simulink model "singlephasesinePWMinverter"  (R2012b)
settings: Solver=ode45  StartTime=0.0  StopTime=1  RelTol=1e-3
libraries: powerlib x7, powerlib_extras x1
settings Model: Creator=Tran Minh Luan  LastModifiedBy=Tran Minh Luan
settings SolverCC: PositivePriorityOrder=on

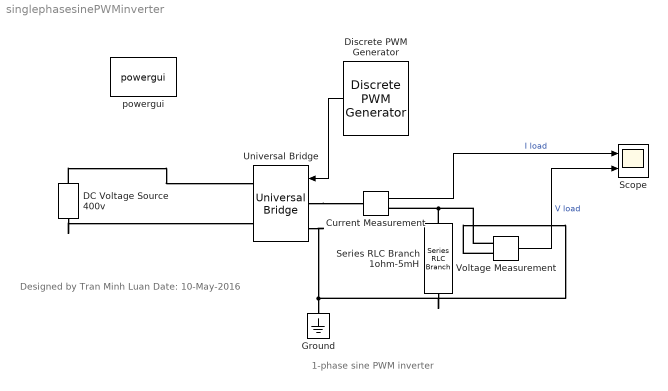
== system singlephasesinePWMinverter ==
  note: Designed by Tran Minh Luan
      | Date: 10-May-2016
  note: 1-phase sine PWM inverter
  Current Measurement : powerlib/Measurements/Current Measurement  PhasorSimulation=off  OutputType=Complex  PSBequivalent=0
  DC Voltage Source 400v : powerlib/Electrical Sources/DC Voltage Source  Amplitude=400  Measurements=None
  Discrete PWM Generator : powerlib_extras/Discrete  Control Blocks/Discrete PWM Generator  GeneratorMode="2-arm  bridge (4 pulses)"  Fc=1080  Ts=5e-6  Internal=on  mIndex=0.8  Freq=60  Phase=0
  Ground : powerlib/Elements/Ground  LConnTagsString=a
  Scope : Scope  NumInputPorts=2
      settings: YMin=-5~-450  YMax=5~450  SaveName=singlephaseSPWMinv
  Series RLC Branch 1ohm-5mH : powerlib/Elements/Series RLC Branch  LConnTagsString=__new0  RConnTagsString=__new0  BranchType=RL  Resistance=1  Inductance=0.005  SetiL0=off  InitialCurrent=0  Capacitance=1e-6  Setx0=off  InitialVoltage=0  Measurements=None
  Universal Bridge : powerlib/Power Electronics/Universal Bridge  Arms=2  SnubberResistance=1e5  SnubberCapacitance=inf  Device=IGBT / Diodes  Ron=1e-5  Lon=0  ForwardVoltages="[  0  0  ]"  ForwardVoltage=0  GTOparameters=[ 10e-6 , 20e-6 ]  IGBTparameters=[ 1e-6 , 2e-6 ]  Measurements=None  Measurements_2=None  converterType=Rectifier
  Voltage Measurement : powerlib/Measurements/Voltage Measurement  PhasorSimulation=off  OutputType=Complex  PSBequivalent=0
  powergui : powerlib/powergui  Priority=1  SimulationMode=Discrete  SolverType=Tustin  SampleTime=5e-6  frequency=60  SPID=off  DisableSnubberDevices=off  DisableRonSwitches=off  DisableVfSwitches=off  SwTol=0  Interpol=off  DisplayEquations=off  FunctionMessages=off  frequencyindice=0  Pbase=100e6  ErrMax=1e-4  Iterations=50  UnitsV=kV  UnitsW=MW  echomessages=off  HookPort=off  EnableUseOfTLC=off  x0status=blocks  RestoreLinks=warning  ResistiveCurrentMeasurement=off  Ylog=off  Xlog=on  ShowGrid=off  save=off  variable=ZData  structure=singlephaseSPWMinv  ZoomFFT=off  StartTime=0.98  cycles=1  DisplayStyle=1  fundamental=60  FreqAxis=off  MaxFrequency=1000  frequencyindicesteady=1  display=off  methode=off
  wires:
  Discrete PWM Generator/1 -> Universal Bridge/1
  Voltage Measurement/1 -> Scope/2  "V load"
  Current Measurement/1 -> Scope/1  "I load"
  connections:
  DC Voltage Source 400v/LConn1 -- Universal Bridge/RConn2
  DC Voltage Source 400v/RConn1 -- Universal Bridge/RConn1
  Universal Bridge/LConn2 -- Voltage Measurement/LConn2 -- Series RLC Branch 1ohm-5mH/RConn1 -- Ground/LConn1
  Universal Bridge/LConn1 -- Current Measurement/LConn1
  Series RLC Branch 1ohm-5mH/LConn1 -- Voltage Measurement/LConn1 -- Current Measurement/RConn1
